simulink model "deneme"  (R2017b)
settings: Solver=ode45  StartTime=0.0  StopTime=10.0  MaxStep=1e-4  RelTol=1e-3
libraries: powerlib_extras x59, powerlib x57, powerlib_meascontrol x6, simulink x3, re_lib x3
(part 2 of 3)

== system deneme/Inverter Control/Current Ref. Generator ==
  note: evd
  note: evq
  evd : Inport
  evq : Inport  Port=2
  Divide : Product  Inputs=*/
  Divide1 : Product  Inputs=/*
  Scope24 : Scope
  Sum1 : Sum  Inputs=-+|
  Sum3 : Sum  Inputs=|++
  Zd : Gain  Gain=0.4559
  Zd1 : Gain  Gain=0.4559
  Zd^2+Zq^2 : Constant  Value=0.4559^2+0.1824^2
  Zq : Gain  Gain=0.1824
  Zq1 : Gain  Gain=0.1824
  id* : Outport
  iq* : Outport  Port=2
  tag scope: id_ref1=global, iq_ref1=global
  wires:
  Zd/1 -> Sum3/1
  Zq1/1 -> Sum3/2
  Zd1/1 -> Sum1/2
  Zq/1 -> Sum1/1
  Sum3/1 -> Divide/1
  Zd^2+Zq^2/1 -> Divide/2, Divide1/1, Scope24/1
  Sum1/1 -> Divide1/2
  evd/1 -> Zd/1, Zq/1
  evq/1 -> Zd1/1, Zq1/1
  Divide1/1 -> iq*/1, [iq_ref1]
  Divide/1 -> id*/1, [id_ref1]

== system deneme/Inverter Control/Frequency Reference Generator ==
  note: theta
  Constant : Constant  Value=2*pi
  Integrator : Integrator  ExternalReset=rising
  Relational Operator : RelationalOperator  OutDataTypeStr=boolean  RndMeth=Nearest
  "f* " : Constant  Value=50
  w* : Gain  Gain=2*pi
  theta* : Outport
  tag scope: f_ref=global, theta=global
  wires:
  "f* "/1 -> w*/1, [f_ref]
  w*/1 -> Integrator/1
  Relational Operator/1 -> Integrator/2
  Constant/1 -> Relational Operator/2
  Integrator/1 -> Relational Operator/1, theta*/1, [theta]

== system deneme/Inverter Control/Iabc  - idq ==
  Iabc : Inport
  theta : Inport  Port=2
  Demux : Demux  Outputs=2
  abc  - alfa/beta : Subsystem
  alfa/beta - dq : Subsystem
  iq : Outport
  id : Outport  Port=2
  tag scope: id1=global, iq1=global
  wires:
  theta/1 -> alfa/beta - dq/2(theta)
  Iabc/1 -> abc  - alfa/beta/1(abc)
  abc  - alfa/beta/1(alfa/beta) -> alfa/beta - dq/1(alfa/beta)
  alfa/beta - dq/1(d/q) -> Demux/1
  Demux/1 -> id/1, [id1]
  Demux/2 -> iq/1, [iq1]

== system deneme/Inverter Control/PI id ==
  e : Inport
  Gain1 : Gain  Gain=50
  Gain2 : Gain  Gain=500
  Integrator : Integrator
  Saturation : Saturate  UpperLimit=inf  LowerLimit=-inf
  Sum1 : Sum  Inputs=|++
  " " : Outport
  wires:
  Sum1/1 -> Saturation/1
  Integrator/1 -> Sum1/2
  Gain1/1 -> Sum1/1
  e/1 -> Gain2/1, Gain1/1
  Gain2/1 -> Integrator/1
  Saturation/1 -> " "/1

== system deneme/Inverter Control/PI iq ==
  e : Inport
  Gain1 : Gain  Gain=50
  Gain2 : Gain  Gain=500
  Integrator : Integrator
  Saturation : Saturate  UpperLimit=inf  LowerLimit=-inf
  Sum1 : Sum  Inputs=|++
  " " : Outport
  wires:
  Saturation/1 -> " "/1
  Gain2/1 -> Integrator/1
  e/1 -> Gain1/1, Gain2/1
  Gain1/1 -> Sum1/1
  Integrator/1 -> Sum1/2
  Sum1/1 -> Saturation/1

== system deneme/Inverter Control/PI vd ==
  e : Inport
  Gain1 : Gain  Gain=2
  Gain2 : Gain  Gain=20
  Integrator : Integrator
  Saturation : Saturate  UpperLimit=inf  LowerLimit=-inf
  Sum1 : Sum  Inputs=|++
  " " : Outport
  wires:
  Saturation/1 -> " "/1
  Gain2/1 -> Integrator/1
  e/1 -> Gain1/1, Gain2/1
  Gain1/1 -> Sum1/1
  Integrator/1 -> Sum1/2
  Sum1/1 -> Saturation/1

== system deneme/Inverter Control/PI vq ==
  e : Inport
  Gain1 : Gain  Gain=2
  Gain2 : Gain  Gain=2
  Integrator : Integrator
  Saturation : Saturate  UpperLimit=inf  LowerLimit=-inf
  Sum1 : Sum  Inputs=|++
  " " : Outport
  wires:
  Sum1/1 -> Saturation/1
  Integrator/1 -> Sum1/2
  Gain1/1 -> Sum1/1
  e/1 -> Gain2/1, Gain1/1
  Gain2/1 -> Integrator/1
  Saturation/1 -> " "/1

== system deneme/Inverter Control/PWM ==
  Uabc_ref : Inport
  Gain2 : Gain  Gain=2/1000
  PWM Generator : powerlib_extras/Control  Blocks/PWM Generator  GeneratorMode="3-arm  bridge (6 pulses)"  Fc=10000  Internal=off  mIndex=0.4  Freq=60  Phase=0
  S : Outport
  tag scope: m_index1=global, pulses1=global
  wires:
  PWM Generator/1 -> S/1, [pulses1]
  Uabc_ref/1 -> Gain2/1
  Gain2/1 -> PWM Generator/1, [m_index1]

== system deneme/Inverter Control/Vabc  - vdq ==
  Vabc : Inport
  theta : Inport  Port=2
  Demux : Demux  Outputs=2
  abc  - alfa/beta : Subsystem
  alfa/beta - dq : Subsystem
  vq : Outport
  vd : Outport  Port=2
  tag scope: vd1=global, vq1=global
  wires:
  Demux/2 -> vq/1, [vq1]
  Demux/1 -> vd/1, [vd1]
  alfa/beta - dq/1(d/q) -> Demux/1
  abc  - alfa/beta/1(alfa/beta) -> alfa/beta - dq/1(alfa/beta)
  Vabc/1 -> abc  - alfa/beta/1(abc)
  theta/1 -> alfa/beta - dq/2(theta)

== system deneme/Inverter Control/vdq - Vabc ==
  Ud/Uq : Inport
  theta : Inport  Port=2
  alfa/beta - abc : Subsystem
  d/q - alfa/beta : Subsystem
  Uabc_ref : Outport
  wires:
  d/q - alfa/beta/1(alfa/beta) -> alfa/beta - abc/1(alfa/beta)
  Ud/Uq/1 -> d/q - alfa/beta/1(d/q)
  alfa/beta - abc/1(abc) -> Uabc_ref/1
  theta/1 -> d/q - alfa/beta/2(tita)

== system deneme/Inverter Control1/ Voltage Reference Generator ==
  Mux4 : Mux  Inputs=3
  Phase A reference : Sin  Amplitude=400*sqrt(2)/sqrt(3)  Frequency=2*pi*50  SampleTime=0
  Phase B reference : Sin  Amplitude=400*sqrt(2)/sqrt(3)  Frequency=2*pi*50  Phase=-2*pi/3  SampleTime=0
  Phase C reference : Sin  Amplitude=400*sqrt(2)/sqrt(3)  Frequency=2*pi*50  Phase=2*pi/3  SampleTime=0
  Product : Product  RndMeth=Zero
  Ramp : simulink/Sources/Ramp  slope=1/0.3  start=0  X0=0
  Saturation : Saturate  UpperLimit=1  LowerLimit=0
  Vabc* : Outport
  tag scope: Vabc_ref2=global
  wires:
  Phase B reference/1 -> Mux4/2
  Phase A reference/1 -> Mux4/1
  Phase C reference/1 -> Mux4/3
  Ramp/1 -> Saturation/1
  Saturation/1 -> Product/2
  Mux4/1 -> Vabc*/1, [Vabc_ref2]

== system deneme/Inverter Control1/Cross Terms ==
  id* : Inport
  iq* : Inport  Port=2
  Gain1 : Gain  Gain=-2*pi*50*3e-3
  Gain2 : Gain  Gain=2*pi*50*3e-3
  " q" : Outport
  " d" : Outport  Port=2
  wires:
  id*/1 -> Gain1/1
  iq*/1 -> Gain2/1
  Gain1/1 -> " d"/1
  Gain2/1 -> " q"/1

== system deneme/Inverter Control1/Current Ref. Generator ==
  note: evd
  note: evq
  evd : Inport
  evq : Inport  Port=2
  Divide : Product  Inputs=*/
  Divide1 : Product  Inputs=/*
  Scope24 : Scope
  Sum1 : Sum  Inputs=-+|
  Sum3 : Sum  Inputs=|++
  Zd : Gain  Gain=0.4559
  Zd1 : Gain  Gain=0.4559
  Zd^2+Zq^2 : Constant  Value=0.4559^2+0.1824^2
  Zq : Gain  Gain=0.1824
  Zq1 : Gain  Gain=0.1824
  id* : Outport
  iq* : Outport  Port=2
  tag scope: id_ref2=global, iq_ref2=global
  wires:
  Zd/1 -> Sum3/1
  Zq1/1 -> Sum3/2
  Zd1/1 -> Sum1/2
  Zq/1 -> Sum1/1
  Sum3/1 -> Divide/1
  Zd^2+Zq^2/1 -> Divide/2, Divide1/1, Scope24/1
  Sum1/1 -> Divide1/2
  evd/1 -> Zd/1, Zq/1
  evq/1 -> Zd1/1, Zq1/1
  Divide1/1 -> iq*/1, [iq_ref2]
  Divide/1 -> id*/1, [id_ref2]

== system deneme/Inverter Control1/Frequency Reference Generator ==
  note: theta
  Constant : Constant  Value=2*pi
  Integrator : Integrator  ExternalReset=rising
  Relational Operator : RelationalOperator  OutDataTypeStr=boolean  RndMeth=Nearest
  "f* " : Constant  Value=50
  w* : Gain  Gain=2*pi
  theta* : Outport
  wires:
  "f* "/1 -> w*/1
  w*/1 -> Integrator/1
  Relational Operator/1 -> Integrator/2
  Constant/1 -> Relational Operator/2
  Integrator/1 -> Relational Operator/1, theta*/1

== system deneme/Inverter Control1/Iabc  - idq ==
  Iabc : Inport
  theta : Inport  Port=2
  Demux : Demux  Outputs=2
  abc  - alfa/beta : Subsystem
  alfa/beta - dq : Subsystem
  iq : Outport
  id : Outport  Port=2
  tag scope: id2=global, iq2=global
  wires:
  theta/1 -> alfa/beta - dq/2(theta)
  Iabc/1 -> abc  - alfa/beta/1(abc)
  abc  - alfa/beta/1(alfa/beta) -> alfa/beta - dq/1(alfa/beta)
  alfa/beta - dq/1(d/q) -> Demux/1
  Demux/1 -> id/1, [id2]
  Demux/2 -> iq/1, [iq2]

== system deneme/Inverter Control1/PI id ==
  e : Inport
  Gain1 : Gain  Gain=50
  Gain2 : Gain  Gain=500
  Integrator : Integrator
  Saturation : Saturate  UpperLimit=inf  LowerLimit=-inf
  Sum1 : Sum  Inputs=|++
  " " : Outport
  wires:
  Sum1/1 -> Saturation/1
  Integrator/1 -> Sum1/2
  Gain1/1 -> Sum1/1
  e/1 -> Gain2/1, Gain1/1
  Gain2/1 -> Integrator/1
  Saturation/1 -> " "/1

== system deneme/Inverter Control1/PI iq ==
  e : Inport
  Gain1 : Gain  Gain=50
  Gain2 : Gain  Gain=500
  Integrator : Integrator
  Saturation : Saturate  UpperLimit=inf  LowerLimit=-inf
  Sum1 : Sum  Inputs=|++
  " " : Outport
  wires:
  Saturation/1 -> " "/1
  Gain2/1 -> Integrator/1
  e/1 -> Gain1/1, Gain2/1
  Gain1/1 -> Sum1/1
  Integrator/1 -> Sum1/2
  Sum1/1 -> Saturation/1

== system deneme/Inverter Control1/PI vd ==
  e : Inport
  Gain1 : Gain  Gain=2
  Gain2 : Gain  Gain=20
  Integrator : Integrator
  Saturation : Saturate  UpperLimit=inf  LowerLimit=-inf
  Sum1 : Sum  Inputs=|++
  " " : Outport
  wires:
  Saturation/1 -> " "/1
  Gain2/1 -> Integrator/1
  e/1 -> Gain1/1, Gain2/1
  Gain1/1 -> Sum1/1
  Integrator/1 -> Sum1/2
  Sum1/1 -> Saturation/1

== system deneme/Inverter Control1/PI vq ==
  e : Inport
  Gain1 : Gain  Gain=2
  Gain2 : Gain  Gain=2
  Integrator : Integrator
  Saturation : Saturate  UpperLimit=inf  LowerLimit=-inf
  Sum1 : Sum  Inputs=|++
  " " : Outport
  wires:
  Sum1/1 -> Saturation/1
  Integrator/1 -> Sum1/2
  Gain1/1 -> Sum1/1
  e/1 -> Gain2/1, Gain1/1
  Gain2/1 -> Integrator/1
  Saturation/1 -> " "/1

== system deneme/Inverter Control1/PWM ==
  Uabc_ref : Inport
  Gain2 : Gain  Gain=2/1000
  PWM Generator : powerlib_extras/Control  Blocks/PWM Generator  GeneratorMode="3-arm  bridge (6 pulses)"  Fc=10000  Internal=off  mIndex=0.4  Freq=60  Phase=0
  S : Outport
  tag scope: m_index2=global, pulses2=global
  wires:
  PWM Generator/1 -> S/1, [pulses2]
  Uabc_ref/1 -> Gain2/1
  Gain2/1 -> PWM Generator/1, [m_index2]

== system deneme/Inverter Control1/Vabc  - vdq ==
  Vabc : Inport
  theta : Inport  Port=2
  Demux : Demux  Outputs=2
  abc  - alfa/beta : Subsystem
  alfa/beta - dq : Subsystem
  vq : Outport
  vd : Outport  Port=2
  tag scope: vd2=global, vq2=global
  wires:
  Demux/2 -> vq/1, [vq2]
  Demux/1 -> vd/1, [vd2]
  alfa/beta - dq/1(d/q) -> Demux/1
  abc  - alfa/beta/1(alfa/beta) -> alfa/beta - dq/1(alfa/beta)
  Vabc/1 -> abc  - alfa/beta/1(abc)
  theta/1 -> alfa/beta - dq/2(theta)

== system deneme/Inverter Control1/vdq - Vabc ==
  Ud/Uq : Inport
  theta : Inport  Port=2
  alfa/beta - abc : Subsystem
  d/q - alfa/beta : Subsystem
  Uabc_ref : Outport
  wires:
  d/q - alfa/beta/1(alfa/beta) -> alfa/beta - abc/1(alfa/beta)
  Ud/Uq/1 -> d/q - alfa/beta/1(d/q)
  alfa/beta - abc/1(abc) -> Uabc_ref/1
  theta/1 -> d/q - alfa/beta/2(tita)

== system deneme/Inverter Control2/ Voltage Reference Generator ==
  Mux4 : Mux  Inputs=3
  Phase A reference : Sin  Amplitude=400*sqrt(2)/sqrt(3)  Frequency=2*pi*50  SampleTime=0
  Phase B reference : Sin  Amplitude=400*sqrt(2)/sqrt(3)  Frequency=2*pi*50  Phase=-2*pi/3  SampleTime=0
  Phase C reference : Sin  Amplitude=400*sqrt(2)/sqrt(3)  Frequency=2*pi*50  Phase=2*pi/3  SampleTime=0
  Product : Product  RndMeth=Zero
  Ramp : simulink/Sources/Ramp  slope=1/0.3  start=0  X0=0
  Saturation : Saturate  UpperLimit=1  LowerLimit=0
  Vabc* : Outport
  tag scope: Vabc_ref3=global
  wires:
  Phase B reference/1 -> Mux4/2
  Phase A reference/1 -> Mux4/1
  Phase C reference/1 -> Mux4/3
  Ramp/1 -> Saturation/1
  Saturation/1 -> Product/2
  Mux4/1 -> Vabc*/1, [Vabc_ref3]

== system deneme/Inverter Control2/Cross Terms ==
  id* : Inport
  iq* : Inport  Port=2
  Gain1 : Gain  Gain=-2*pi*50*3e-3
  Gain2 : Gain  Gain=2*pi*50*3e-3
  " q" : Outport
  " d" : Outport  Port=2
  wires:
  id*/1 -> Gain1/1
  iq*/1 -> Gain2/1
  Gain1/1 -> " d"/1
  Gain2/1 -> " q"/1

== system deneme/Inverter Control2/Current Ref. Generator ==
  note: evd
  note: evq
  evd : Inport
  evq : Inport  Port=2
  Divide : Product  Inputs=*/
  Divide1 : Product  Inputs=/*
  Scope24 : Scope
  Sum1 : Sum  Inputs=-+|
  Sum3 : Sum  Inputs=|++
  Zd : Gain  Gain=0.4559
  Zd1 : Gain  Gain=0.4559
  Zd^2+Zq^2 : Constant  Value=0.4559^2+0.1824^2
  Zq : Gain  Gain=0.1824
  Zq1 : Gain  Gain=0.1824
  id* : Outport
  iq* : Outport  Port=2
  tag scope: id_ref3=global, iq_ref3=global
  wires:
  Zd/1 -> Sum3/1
  Zq1/1 -> Sum3/2
  Zd1/1 -> Sum1/2
  Zq/1 -> Sum1/1
  Sum3/1 -> Divide/1
  Zd^2+Zq^2/1 -> Divide/2, Divide1/1, Scope24/1
  Sum1/1 -> Divide1/2
  evd/1 -> Zd/1, Zq/1
  evq/1 -> Zd1/1, Zq1/1
  Divide1/1 -> iq*/1, [iq_ref3]
  Divide/1 -> id*/1, [id_ref3]

== system deneme/Inverter Control2/Frequency Reference Generator ==
  note: theta
  Constant : Constant  Value=2*pi
  Integrator : Integrator  ExternalReset=rising
  Relational Operator : RelationalOperator  OutDataTypeStr=boolean  RndMeth=Nearest
  "f* " : Constant  Value=50
  w* : Gain  Gain=2*pi
  theta* : Outport
  wires:
  "f* "/1 -> w*/1
  w*/1 -> Integrator/1
  Relational Operator/1 -> Integrator/2
  Constant/1 -> Relational Operator/2
  Integrator/1 -> Relational Operator/1, theta*/1

== system deneme/Inverter Control2/Iabc  - idq ==
  Iabc : Inport
  theta : Inport  Port=2
  Demux : Demux  Outputs=2
  abc  - alfa/beta : Subsystem
  alfa/beta - dq : Subsystem
  iq : Outport
  id : Outport  Port=2
  tag scope: id3=global, iq3=global
  wires:
  theta/1 -> alfa/beta - dq/2(theta)
  Iabc/1 -> abc  - alfa/beta/1(abc)
  abc  - alfa/beta/1(alfa/beta) -> alfa/beta - dq/1(alfa/beta)
  alfa/beta - dq/1(d/q) -> Demux/1
  Demux/1 -> id/1, [id3]
  Demux/2 -> iq/1, [iq3]

== system deneme/Inverter Control2/PI id ==
  e : Inport
  Gain1 : Gain  Gain=50
  Gain2 : Gain  Gain=500
  Integrator : Integrator
  Saturation : Saturate  UpperLimit=inf  LowerLimit=-inf
  Sum1 : Sum  Inputs=|++
  " " : Outport
  wires:
  Sum1/1 -> Saturation/1
  Integrator/1 -> Sum1/2
  Gain1/1 -> Sum1/1
  e/1 -> Gain2/1, Gain1/1
  Gain2/1 -> Integrator/1
  Saturation/1 -> " "/1

== system deneme/Inverter Control2/PI iq ==
  e : Inport
  Gain1 : Gain  Gain=50
  Gain2 : Gain  Gain=500
  Integrator : Integrator
  Saturation : Saturate  UpperLimit=inf  LowerLimit=-inf
  Sum1 : Sum  Inputs=|++
  " " : Outport
  wires:
  Saturation/1 -> " "/1
  Gain2/1 -> Integrator/1
  e/1 -> Gain1/1, Gain2/1
  Gain1/1 -> Sum1/1
  Integrator/1 -> Sum1/2
  Sum1/1 -> Saturation/1

== system deneme/Inverter Control2/PI vd ==
  e : Inport
  Gain1 : Gain  Gain=2
  Gain2 : Gain  Gain=20
  Integrator : Integrator
  Saturation : Saturate  UpperLimit=inf  LowerLimit=-inf
  Sum1 : Sum  Inputs=|++
  " " : Outport
  wires:
  Saturation/1 -> " "/1
  Gain2/1 -> Integrator/1
  e/1 -> Gain1/1, Gain2/1
  Gain1/1 -> Sum1/1
  Integrator/1 -> Sum1/2
  Sum1/1 -> Saturation/1

== system deneme/Inverter Control2/PI vq ==
  e : Inport
  Gain1 : Gain  Gain=2
  Gain2 : Gain  Gain=2
  Integrator : Integrator
  Saturation : Saturate  UpperLimit=inf  LowerLimit=-inf
  Sum1 : Sum  Inputs=|++
  " " : Outport
  wires:
  Sum1/1 -> Saturation/1
  Integrator/1 -> Sum1/2
  Gain1/1 -> Sum1/1
  e/1 -> Gain2/1, Gain1/1
  Gain2/1 -> Integrator/1
  Saturation/1 -> " "/1

== system deneme/Inverter Control2/PWM ==
  Uabc_ref : Inport
  Gain2 : Gain  Gain=2/1000
  PWM Generator : powerlib_extras/Control  Blocks/PWM Generator  GeneratorMode="3-arm  bridge (6 pulses)"  Fc=10000  Internal=off  mIndex=0.4  Freq=60  Phase=0
  S : Outport
  tag scope: m_index3=global, pulses3=global
  wires:
  PWM Generator/1 -> S/1, [pulses3]
  Uabc_ref/1 -> Gain2/1
  Gain2/1 -> PWM Generator/1, [m_index3]

== system deneme/Inverter Control2/Vabc  - vdq ==
  Vabc : Inport
  theta : Inport  Port=2
  Demux : Demux  Outputs=2
  abc  - alfa/beta : Subsystem
  alfa/beta - dq : Subsystem
  vq : Outport
  vd : Outport  Port=2
  tag scope: vd3=global, vq3=global
  wires:
  Demux/2 -> vq/1, [vq3]
  Demux/1 -> vd/1, [vd3]
  alfa/beta - dq/1(d/q) -> Demux/1
  abc  - alfa/beta/1(alfa/beta) -> alfa/beta - dq/1(alfa/beta)
  Vabc/1 -> abc  - alfa/beta/1(abc)
  theta/1 -> alfa/beta - dq/2(theta)

== system deneme/Inverter Control2/vdq - Vabc ==
  Ud/Uq : Inport
  theta : Inport  Port=2
  alfa/beta - abc : Subsystem
  d/q - alfa/beta : Subsystem
  Uabc_ref : Outport
  wires:
  d/q - alfa/beta/1(alfa/beta) -> alfa/beta - abc/1(alfa/beta)
  Ud/Uq/1 -> d/q - alfa/beta/1(d/q)
  alfa/beta - abc/1(abc) -> Uabc_ref/1
  theta/1 -> d/q - alfa/beta/2(tita)

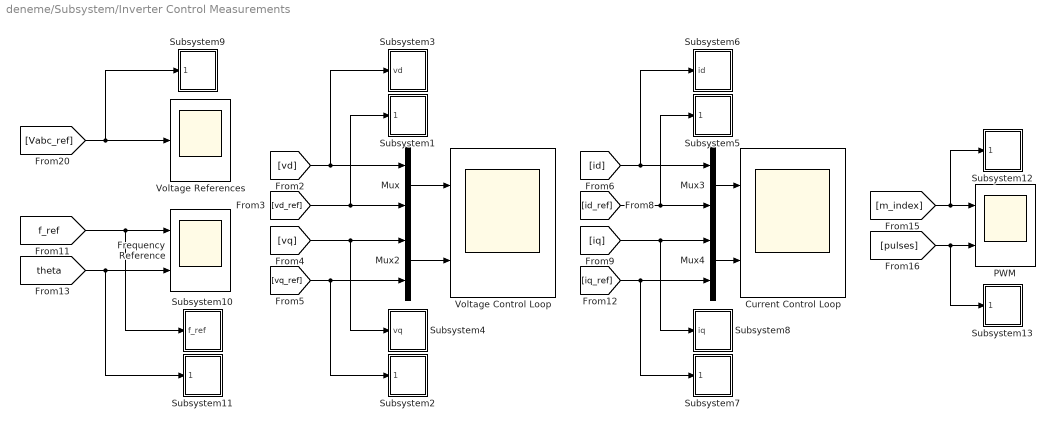
== system deneme/Subsystem/Inverter Control Measurements ==
  Current Control Loop : Scope  NumInputPorts=2
  Frequency Reference : Scope  NumInputPorts=2
  Mux{,2..4} (4 alike) : Mux  Inputs=2
  PWM : Scope  NumInputPorts=2
  Subsystem1 : Subsystem
  Subsystem10 : Subsystem
  Subsystem11 : Subsystem
  Subsystem12 : Subsystem
  Subsystem13 : Subsystem
  Subsystem2 : Subsystem
  Subsystem3 : Subsystem
  Subsystem4 : Subsystem
  Subsystem5 : Subsystem
  Subsystem6 : Subsystem
  Subsystem7 : Subsystem
  Subsystem8 : Subsystem
  Subsystem9 : Subsystem
  Voltage Control Loop : Scope  NumInputPorts=2
  Voltage References : Scope
  wires:
  [vd] -> Mux/1, Subsystem3/1(vd)
  [vd_ref] -> Mux/2, Subsystem1/1(vd_ref)
  [vq] -> Mux2/1, Subsystem4/1(vq)
  [vq_ref] -> Mux2/2, Subsystem2/1(vq_ref)
  Mux/1 -> Voltage Control Loop/1
  Mux2/1 -> Voltage Control Loop/2
  [id] -> Mux3/1, Subsystem6/1(id)
  [id_ref] -> Mux3/2, Subsystem5/1(id_ref)
  [iq] -> Mux4/1, Subsystem8/1(iq)
  [iq_ref] -> Mux4/2, Subsystem7/1(iq_ref)
  [Vabc_ref] -> Voltage References/1, Subsystem9/1(Vabc_ref)
  Mux3/1 -> Current Control Loop/1
  Mux4/1 -> Current Control Loop/2
  [theta] -> Frequency Reference/2, Subsystem11/1(theta)
  [f_ref] -> Frequency Reference/1, Subsystem10/1(f_ref)
  [pulses] -> PWM/2, Subsystem13/1(pulses)
  [m_index] -> PWM/1, Subsystem12/1(m_index)

== system deneme/Subsystem/Inverter Control Measurements1 ==
  Boost Converter Control MPPT : Scope  NumInputPorts=3
  wires:
  [Vref] -> Boost Converter Control MPPT/1
  [delta] -> Boost Converter Control MPPT/2
  [pulsos] -> Boost Converter Control MPPT/3

== system deneme/Subsystem/Inverter Control Measurements2 ==
  Control Loops : Scope  NumInputPorts=2
  Mux : Mux  Inputs=2
  Mux2 : Mux  Inputs=2
  Switch Control : Scope  NumInputPorts=3
  wires:
  [Vdc] -> Mux/1
  [Vdc_ref] -> Mux/2
  [Ibat] -> Mux2/1
  [Ibat_ref] -> Mux2/2
  Mux/1 -> Control Loops/1
  Mux2/1 -> Control Loops/2
  [Sign] -> Switch Control/1
  [S1] -> Switch Control/2
  [S2] -> Switch Control/3

== system deneme/Subsystem/Inverter Control Measurements3 ==
  PLL : Subsystem
  Subsystem : Subsystem
  wires:
  Subsystem/1(Vabc) -> PLL/1(Vabc)

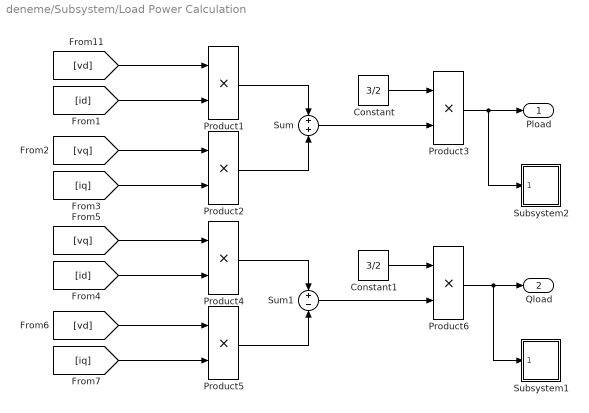
== system deneme/Subsystem/Load Power Calculation ==
  Constant : Constant  Value=3/2
  Constant1 : Constant  Value=3/2
  Product{1..6} (6 alike) : Product  RndMeth=Zero
  Subsystem1 : Subsystem
  Subsystem2 : Subsystem
  Sum : Sum  Inputs=+|+
  Sum1 : Sum  Inputs=+|-
  Pload : Outport
  Qload : Outport  Port=2
  wires:
  [vd] -> Product1/1
  [id] -> Product1/2
  [vq] -> Product2/1
  [iq] -> Product2/2
  Product1/1 -> Sum/1
  Product2/1 -> Sum/2
  Sum/1 -> Product3/2
  Constant/1 -> Product3/1
  Product3/1 -> Pload/1, Subsystem2/1(Pload)
  [vq] -> Product4/1
  [id] -> Product4/2
  [vd] -> Product5/1
  [iq] -> Product5/2
  Product4/1 -> Sum1/1
  Product5/1 -> Sum1/2
  Sum1/1 -> Product6/2
  Constant1/1 -> Product6/1
  Product6/1 -> Qload/1, Subsystem1/1(Qacload)

== system deneme/Subsystem/Subsystem ==
  Mux : Mux  Inputs=3
  Vabc : Outport
  wires:
  Mux/1 -> Vabc/1
  [Vab] -> Mux/1
  [Vbc] -> Mux/2
  [Vca] -> Mux/3

== system deneme/Subsystem/Subsystem1 ==
  Pbus : Inport
  LPF vq11 : powerlib_extras/Discrete  Control Blocks/Discrete 1st-Order Filter  FilterType=Lowpass  Tc=10e-3  Ts=5e-6  Initialize=off  Vac_Init=[0.8 -25 60]  Vdc_Init=0  PlotResponse=off  param1=[1 100 0.1]
  To Workspace1 : ToWorkspace  VariableName=Pbus  SampleTime=-1
  To Workspace2 : ToWorkspace  VariableName=Pbus1  SampleTime=-1
  tag scope: Pbus=global
  wires:
  Pbus/1 -> [Pbus], To Workspace1/1, LPF vq11/1
  LPF vq11/1 -> To Workspace2/1

== system deneme/Subsystem/Subsystem10 ==
  f : Inport
  LPF vq7 : powerlib_extras/Discrete  Control Blocks/Discrete 1st-Order Filter  FilterType=Lowpass  Tc=10e-3  Ts=5e-6  Initialize=off  Vac_Init=[0.8 -25 60]  Vdc_Init=0  PlotResponse=off  param1=[1 100 0.1]
  To Workspace1 : ToWorkspace  VariableName=fabc_real  SampleTime=-1
  To Workspace2 : ToWorkspace  VariableName=fabc_real_fil  SampleTime=-1
  Zero-Order Hold : ZeroOrderHold  SampleTime=5e-6
  wires:
  f/1 -> Zero-Order Hold/1
  LPF vq7/1 -> To Workspace2/1
  Zero-Order Hold/1 -> To Workspace1/1, LPF vq7/1

== system deneme/Subsystem/Subsystem11 ==
  LPF vq{2..3,8..9} (4 alike) : powerlib_extras/Discrete  Control Blocks/Discrete 1st-Order Filter  FilterType=Lowpass  Tc=10e-3  Ts=5e-6  Initialize=off  Vac_Init=[0.8 -25 60]  Vdc_Init=0  PlotResponse=off  param1=[1 100 0.1]
  Load Measurements1 : Scope  NumInputPorts=2
  Load Measurements3 : Scope  NumInputPorts=2
  Load Power Calculation1 : Subsystem
  Load Power Calculation2 : Subsystem
  Load Powers1 : Scope  NumInputPorts=2
  Load Powers2 : Scope  NumInputPorts=2
  wires:
  [Vabc2] -> Load Measurements1/1
  [Iabc2] -> Load Measurements1/2
  Load Power Calculation1/1(Pload) -> LPF vq2/1
  Load Power Calculation1/2(Qload) -> LPF vq3/1
  LPF vq2/1 -> Load Powers1/1
  LPF vq3/1 -> Load Powers1/2
  [Vabc3] -> Load Measurements3/1
  [Iabc3] -> Load Measurements3/2
  Load Power Calculation2/1(Pload) -> LPF vq8/1
  Load Power Calculation2/2(Qload) -> LPF vq9/1
  LPF vq8/1 -> Load Powers2/1
  LPF vq9/1 -> Load Powers2/2

== system deneme/Subsystem/Subsystem3 ==
  Pdc : Inport
  LPF vq7 : powerlib_extras/Discrete  Control Blocks/Discrete 1st-Order Filter  FilterType=Lowpass  Tc=10e-3  Ts=5e-6  Initialize=off  Vac_Init=[0.8 -25 60]  Vdc_Init=0  PlotResponse=off  param1=[1 100 0.1]
  To Workspace1 : ToWorkspace  VariableName=Pdc  SampleTime=-1
  To Workspace2 : ToWorkspace  VariableName=Pdc1  SampleTime=-1
  tag scope: Pdc=global
  wires:
  Pdc/1 -> [Pdc], To Workspace1/1, LPF vq7/1
  LPF vq7/1 -> To Workspace2/1

== system deneme/Subsystem/Subsystem4 ==
  Ppv : Inport
  LPF vq7 : powerlib_extras/Discrete  Control Blocks/Discrete 1st-Order Filter  FilterType=Lowpass  Tc=10e-3  Ts=5e-6  Initialize=off  Vac_Init=[0.8 -25 60]  Vdc_Init=0  PlotResponse=off  param1=[1 100 0.1]
  To Workspace1 : ToWorkspace  VariableName=Ppv  SampleTime=-1
  To Workspace2 : ToWorkspace  VariableName=Ppv1  SampleTime=-1
  tag scope: Ppv=global
  wires:
  Ppv/1 -> [Ppv], To Workspace1/1, LPF vq7/1
  LPF vq7/1 -> To Workspace2/1

== system deneme/Subsystem/Subsystem5 ==
  Pbat : Inport
  LPF vq7 : powerlib_extras/Discrete  Control Blocks/Discrete 1st-Order Filter  FilterType=Lowpass  Tc=10e-3  Ts=5e-6  Initialize=off  Vac_Init=[0.8 -25 60]  Vdc_Init=0  PlotResponse=off  param1=[1 100 0.1]
  To Workspace1 : ToWorkspace  VariableName=Pbat  SampleTime=-1
  To Workspace2 : ToWorkspace  VariableName=Pbat1  SampleTime=-1
  tag scope: Pbat=global
  wires:
  Pbat/1 -> [Pbat], To Workspace1/1, LPF vq7/1
  LPF vq7/1 -> To Workspace2/1

== system deneme/Subsystem/Subsystem6 ==
  Vab_rms : Inport
  To Workspace1 : ToWorkspace  VariableName=Vab_rms  SampleTime=-1
  tag scope: Vab_rms=global
  wires:
  Vab_rms/1 -> To Workspace1/1, [Vab_rms]

== system deneme/Subsystem/Subsystem7 ==
  Va_rms : Inport
  To Workspace1 : ToWorkspace  VariableName=Va_rms  SampleTime=-1
  tag scope: Va_rms=global
  wires:
  Va_rms/1 -> [Va_rms], To Workspace1/1

== system deneme/Subsystem/Subsystem8 ==
  Pdcinv : Inport
  LPF vq7 : powerlib_extras/Discrete  Control Blocks/Discrete 1st-Order Filter  FilterType=Lowpass  Tc=10e-3  Ts=5e-6  Initialize=off  Vac_Init=[0.8 -25 60]  Vdc_Init=0  PlotResponse=off  param1=[1 100 0.1]
  To Workspace1 : ToWorkspace  VariableName=Pdcinv  SampleTime=-1
  To Workspace2 : ToWorkspace  VariableName=Pdcinv1  SampleTime=-1
  tag scope: Pdcinv=global
  wires:
  Pdcinv/1 -> [Pdcinv], To Workspace1/1, LPF vq7/1
  LPF vq7/1 -> To Workspace2/1

== system deneme/Subsystem/Subsystem9 ==
  Mux1 : Mux  Inputs=3
  Iabc : Outport
  wires:
  [Ia] -> Mux1/1
  [Ib] -> Mux1/2
  [Ic] -> Mux1/3
  Mux1/1 -> Iabc/1

== system deneme/Boost/Incremental Conductance MPPT/Subsystem1 ==
  Vref : Inport
  To Workspace1 : ToWorkspace  VariableName=Vref  SampleTime=-1
  Zero-Order Hold : ZeroOrderHold  SampleTime=5e-6
  tag scope: Vref=global
  wires:
  Vref/1 -> Zero-Order Hold/1
  Zero-Order Hold/1 -> [Vref], To Workspace1/1

== system deneme/Boost/Incremental Conductance MPPT/Subsystem2 ==
  delta : Inport
  To Workspace1 : ToWorkspace  VariableName=delta  SampleTime=-1
  Zero-Order Hold : ZeroOrderHold  SampleTime=5e-6
  tag scope: delta=global
  wires:
  delta/1 -> Zero-Order Hold/1
  Zero-Order Hold/1 -> To Workspace1/1, [delta]

== system deneme/Boost/Incremental Conductance MPPT/Subsystem3 ==
  pulsos : Inport
  To Workspace1 : ToWorkspace  VariableName=pulsos  SampleTime=-1
  Zero-Order Hold : ZeroOrderHold  SampleTime=5e-6
  tag scope: pulsos=global
  wires:
  pulsos/1 -> Zero-Order Hold/1
  Zero-Order Hold/1 -> [pulsos], To Workspace1/1

== system deneme/Boost1/Incremental Conductance MPPT/Subsystem1 ==
  Vref : Inport
  To Workspace1 : ToWorkspace  VariableName=Vref2  SampleTime=-1
  Zero-Order Hold : ZeroOrderHold  SampleTime=5e-6
  tag scope: Vref2=global
  wires:
  Vref/1 -> Zero-Order Hold/1
  Zero-Order Hold/1 -> To Workspace1/1, [Vref2]

== system deneme/Boost1/Incremental Conductance MPPT/Subsystem2 ==
  delta : Inport
  To Workspace1 : ToWorkspace  VariableName=delta2  SampleTime=-1
  Zero-Order Hold : ZeroOrderHold  SampleTime=5e-6
  tag scope: delta2=global
  wires:
  delta/1 -> Zero-Order Hold/1
  Zero-Order Hold/1 -> To Workspace1/1, [delta2]

== system deneme/Boost1/Incremental Conductance MPPT/Subsystem3 ==
  pulsos : Inport
  To Workspace1 : ToWorkspace  VariableName=pulsos2  SampleTime=-1
  Zero-Order Hold : ZeroOrderHold  SampleTime=5e-6
  tag scope: pulsos2=global
  wires:
  pulsos/1 -> Zero-Order Hold/1
  Zero-Order Hold/1 -> [pulsos2], To Workspace1/1

== system deneme/Boost2/Incremental Conductance MPPT/Subsystem1 ==
  Vref : Inport
  To Workspace1 : ToWorkspace  VariableName=Vref3  SampleTime=-1
  Zero-Order Hold : ZeroOrderHold  SampleTime=5e-6
  tag scope: Vref3=global
  wires:
  Zero-Order Hold/1 -> [Vref3], To Workspace1/1
  Vref/1 -> Zero-Order Hold/1

== system deneme/Boost2/Incremental Conductance MPPT/Subsystem2 ==
  delta : Inport
  To Workspace1 : ToWorkspace  VariableName=delta3  SampleTime=-1
  Zero-Order Hold : ZeroOrderHold  SampleTime=5e-6
  tag scope: delta3=global
  wires:
  Zero-Order Hold/1 -> [delta3], To Workspace1/1
  delta/1 -> Zero-Order Hold/1

== system deneme/Boost2/Incremental Conductance MPPT/Subsystem3 ==
  pulsos : Inport
  To Workspace1 : ToWorkspace  VariableName=pulsos3  SampleTime=-1
  Zero-Order Hold : ZeroOrderHold  SampleTime=5e-6
  tag scope: pulsos3=global
  wires:
  Zero-Order Hold/1 -> To Workspace1/1, [pulsos3]
  pulsos/1 -> Zero-Order Hold/1

== system deneme/Inverter Control/Iabc  - idq/abc  - alfa//beta ==
  abc : Inport
  Mux : Mux  Inputs=2
  d_s : Fcn  Expr=(-1/sqrt(3)*u(2))+(1/sqrt(3)*u(3))
  q_s : Fcn  Expr=(2/3)*u(1)-(1/3)*u(2)-(1/3)*u(3)
  alfa/beta : Outport
  wires:
  abc/1 -> q_s/1, d_s/1
  d_s/1 -> Mux/1
  q_s/1 -> Mux/2
  Mux/1 -> alfa/beta/1

== system deneme/Inverter Control/Iabc  - idq/alfa//beta - dq ==
  alfa/beta : Inport
  theta : Inport  Port=2
  Mux : Mux  Inputs=2
  Mux1 : Mux  Inputs=2
  d : Fcn  Expr=u(2)*sin(u(3)) + u(1)*cos(u(3))
  q : Fcn  Expr=-u(1)*sin(u(3)) + u(2)*cos(u(3))
  d/q : Outport
  wires:
  d/1 -> Mux/1
  q/1 -> Mux/2
  Mux/1 -> d/q/1
  alfa/beta/1 -> Mux1/1
  theta/1 -> Mux1/2
  Mux1/1 -> d/1, q/1

== system deneme/Inverter Control/Vabc  - vdq/abc  - alfa//beta ==
  abc : Inport
  Mux : Mux  Inputs=2
  d_s : Fcn  Expr=(-1/sqrt(3)*u(2))+(1/sqrt(3)*u(3))
  q_s : Fcn  Expr=(2/3)*u(1)-(1/3)*u(2)-(1/3)*u(3)
  alfa/beta : Outport
  wires:
  Mux/1 -> alfa/beta/1
  q_s/1 -> Mux/2
  d_s/1 -> Mux/1
  abc/1 -> d_s/1, q_s/1

== system deneme/Inverter Control/Vabc  - vdq/alfa//beta - dq ==
  alfa/beta : Inport
  theta : Inport  Port=2
  Mux : Mux  Inputs=2
  Mux1 : Mux  Inputs=2
  d : Fcn  Expr=u(2)*sin(u(3)) + u(1)*cos(u(3))
  q : Fcn  Expr=-u(1)*sin(u(3)) + u(2)*cos(u(3))
  d/q : Outport
  wires:
  Mux1/1 -> q/1, d/1
  theta/1 -> Mux1/2
  alfa/beta/1 -> Mux1/1
  Mux/1 -> d/q/1
  q/1 -> Mux/2
  d/1 -> Mux/1

== system deneme/Inverter Control/vdq - Vabc/alfa//beta - abc ==
  alfa/beta : Inport
  Mux : Mux  Inputs=3
  a : Fcn  Expr=u[2]
  b : Fcn  Expr=-sqrt(3)/2*u[1]-0.5*u[2]
  c : Fcn  Expr=sqrt(3)/2*u[1]-0.5*u[2]
  abc : Outport
  tag scope: Vca_ref1=global, Vcb_ref1=global, Vcc_ref1=global
  wires:
  alfa/beta/1 -> c/1, a/1, b/1
  Mux/1 -> abc/1
  c/1 -> Mux/3, [Vcc_ref1]
  b/1 -> Mux/2, [Vcb_ref1]
  a/1 -> Mux/1, [Vca_ref1]

== system deneme/Inverter Control/vdq - Vabc/d//q - alfa//beta ==
  d/q : Inport
  tita : Inport  Port=2
  Mux : Mux  Inputs=2
  Mux1 : Mux  Inputs=2
  a : Fcn  Expr=-u[2]*sin(u[3]) + u[1]*cos(u[3])
  b : Fcn  Expr=u[1]*sin(u[3]) + u[2]*cos(u[3])
  alfa/beta : Outport
  wires:
  Mux1/1 -> b/1, a/1
  tita/1 -> Mux1/2
  d/q/1 -> Mux1/1
  a/1 -> Mux/1
  b/1 -> Mux/2
  Mux/1 -> alfa/beta/1

== system deneme/Inverter Control1/Iabc  - idq/abc  - alfa//beta ==
  abc : Inport
  Mux : Mux  Inputs=2
  d_s : Fcn  Expr=(-1/sqrt(3)*u(2))+(1/sqrt(3)*u(3))
  q_s : Fcn  Expr=(2/3)*u(1)-(1/3)*u(2)-(1/3)*u(3)
  alfa/beta : Outport
  wires:
  abc/1 -> q_s/1, d_s/1
  d_s/1 -> Mux/1
  q_s/1 -> Mux/2
  Mux/1 -> alfa/beta/1

== system deneme/Inverter Control1/Iabc  - idq/alfa//beta - dq ==
  alfa/beta : Inport
  theta : Inport  Port=2
  Mux : Mux  Inputs=2
  Mux1 : Mux  Inputs=2
  d : Fcn  Expr=u(2)*sin(u(3)) + u(1)*cos(u(3))
  q : Fcn  Expr=-u(1)*sin(u(3)) + u(2)*cos(u(3))
  d/q : Outport
  wires:
  d/1 -> Mux/1
  q/1 -> Mux/2
  Mux/1 -> d/q/1
  alfa/beta/1 -> Mux1/1
  theta/1 -> Mux1/2
  Mux1/1 -> d/1, q/1

== system deneme/Inverter Control1/Vabc  - vdq/abc  - alfa//beta ==
  abc : Inport
  Mux : Mux  Inputs=2
  d_s : Fcn  Expr=(-1/sqrt(3)*u(2))+(1/sqrt(3)*u(3))
  q_s : Fcn  Expr=(2/3)*u(1)-(1/3)*u(2)-(1/3)*u(3)
  alfa/beta : Outport
  wires:
  Mux/1 -> alfa/beta/1
  q_s/1 -> Mux/2
  d_s/1 -> Mux/1
  abc/1 -> d_s/1, q_s/1

== system deneme/Inverter Control1/Vabc  - vdq/alfa//beta - dq ==
  alfa/beta : Inport
  theta : Inport  Port=2
  Mux : Mux  Inputs=2
  Mux1 : Mux  Inputs=2
  d : Fcn  Expr=u(2)*sin(u(3)) + u(1)*cos(u(3))
  q : Fcn  Expr=-u(1)*sin(u(3)) + u(2)*cos(u(3))
  d/q : Outport
  wires:
  Mux1/1 -> q/1, d/1
  theta/1 -> Mux1/2
  alfa/beta/1 -> Mux1/1
  Mux/1 -> d/q/1
  q/1 -> Mux/2
  d/1 -> Mux/1

== system deneme/Inverter Control1/vdq - Vabc/alfa//beta - abc ==
  alfa/beta : Inport
  Mux : Mux  Inputs=3
  a : Fcn  Expr=u[2]
  b : Fcn  Expr=-sqrt(3)/2*u[1]-0.5*u[2]
  c : Fcn  Expr=sqrt(3)/2*u[1]-0.5*u[2]
  abc : Outport
  tag scope: Vca_ref2=global, Vcb_ref2=global, Vcc_ref2=global
  wires:
  alfa/beta/1 -> c/1, a/1, b/1
  Mux/1 -> abc/1
  c/1 -> Mux/3, [Vcc_ref2]
  b/1 -> Mux/2, [Vcb_ref2]
  a/1 -> Mux/1, [Vca_ref2]

== system deneme/Inverter Control1/vdq - Vabc/d//q - alfa//beta ==
  d/q : Inport
  tita : Inport  Port=2
  Mux : Mux  Inputs=2
  Mux1 : Mux  Inputs=2
  a : Fcn  Expr=-u[2]*sin(u[3]) + u[1]*cos(u[3])
  b : Fcn  Expr=u[1]*sin(u[3]) + u[2]*cos(u[3])
  alfa/beta : Outport
  wires:
  Mux1/1 -> b/1, a/1
  tita/1 -> Mux1/2
  d/q/1 -> Mux1/1
  a/1 -> Mux/1
  b/1 -> Mux/2
  Mux/1 -> alfa/beta/1

== system deneme/Inverter Control2/Iabc  - idq/abc  - alfa//beta ==
  abc : Inport
  Mux : Mux  Inputs=2
  d_s : Fcn  Expr=(-1/sqrt(3)*u(2))+(1/sqrt(3)*u(3))
  q_s : Fcn  Expr=(2/3)*u(1)-(1/3)*u(2)-(1/3)*u(3)
  alfa/beta : Outport
  wires:
  abc/1 -> q_s/1, d_s/1
  d_s/1 -> Mux/1
  q_s/1 -> Mux/2
  Mux/1 -> alfa/beta/1

== system deneme/Inverter Control2/Iabc  - idq/alfa//beta - dq ==
  alfa/beta : Inport
  theta : Inport  Port=2
  Mux : Mux  Inputs=2
  Mux1 : Mux  Inputs=2
  d : Fcn  Expr=u(2)*sin(u(3)) + u(1)*cos(u(3))
  q : Fcn  Expr=-u(1)*sin(u(3)) + u(2)*cos(u(3))
  d/q : Outport
  wires:
  d/1 -> Mux/1
  q/1 -> Mux/2
  Mux/1 -> d/q/1
  alfa/beta/1 -> Mux1/1
  theta/1 -> Mux1/2
  Mux1/1 -> d/1, q/1

== system deneme/Inverter Control2/Vabc  - vdq/abc  - alfa//beta ==
  abc : Inport
  Mux : Mux  Inputs=2
  d_s : Fcn  Expr=(-1/sqrt(3)*u(2))+(1/sqrt(3)*u(3))
  q_s : Fcn  Expr=(2/3)*u(1)-(1/3)*u(2)-(1/3)*u(3)
  alfa/beta : Outport
  wires:
  Mux/1 -> alfa/beta/1
  q_s/1 -> Mux/2
  d_s/1 -> Mux/1
  abc/1 -> d_s/1, q_s/1

== system deneme/Inverter Control2/Vabc  - vdq/alfa//beta - dq ==
  alfa/beta : Inport
  theta : Inport  Port=2
  Mux : Mux  Inputs=2
  Mux1 : Mux  Inputs=2
  d : Fcn  Expr=u(2)*sin(u(3)) + u(1)*cos(u(3))
  q : Fcn  Expr=-u(1)*sin(u(3)) + u(2)*cos(u(3))
  d/q : Outport
  wires:
  Mux1/1 -> q/1, d/1
  theta/1 -> Mux1/2
  alfa/beta/1 -> Mux1/1
  Mux/1 -> d/q/1
  q/1 -> Mux/2
  d/1 -> Mux/1

== system deneme/Inverter Control2/vdq - Vabc/alfa//beta - abc ==
  alfa/beta : Inport
  Mux : Mux  Inputs=3
  a : Fcn  Expr=u[2]
  b : Fcn  Expr=-sqrt(3)/2*u[1]-0.5*u[2]
  c : Fcn  Expr=sqrt(3)/2*u[1]-0.5*u[2]
  abc : Outport
  tag scope: Vca_ref3=global, Vcb_ref3=global, Vcc_ref3=global
  wires:
  alfa/beta/1 -> c/1, a/1, b/1
  Mux/1 -> abc/1
  c/1 -> Mux/3, [Vcc_ref3]
  b/1 -> Mux/2, [Vcb_ref3]
  a/1 -> Mux/1, [Vca_ref3]

== system deneme/Inverter Control2/vdq - Vabc/d//q - alfa//beta ==
  d/q : Inport
  tita : Inport  Port=2
  Mux : Mux  Inputs=2
  Mux1 : Mux  Inputs=2
  a : Fcn  Expr=-u[2]*sin(u[3]) + u[1]*cos(u[3])
  b : Fcn  Expr=u[1]*sin(u[3]) + u[2]*cos(u[3])
  alfa/beta : Outport
  wires:
  Mux1/1 -> b/1, a/1
  tita/1 -> Mux1/2
  d/q/1 -> Mux1/1
  a/1 -> Mux/1
  b/1 -> Mux/2
  Mux/1 -> alfa/beta/1

== system deneme/Subsystem/Inverter Control Measurements/Subsystem1 ==
  vd_ref : Inport
  To Workspace1 : ToWorkspace  VariableName=vd_ref  SampleTime=-1
  Zero-Order Hold1 : ZeroOrderHold  SampleTime=5e-6
  wires:
  vd_ref/1 -> Zero-Order Hold1/1
  Zero-Order Hold1/1 -> To Workspace1/1

== system deneme/Subsystem/Inverter Control Measurements/Subsystem10 ==
  f_ref : Inport
  To Workspace1 : ToWorkspace  VariableName=f_ref  SampleTime=-1
  Zero-Order Hold1 : ZeroOrderHold  SampleTime=5e-6
  wires:
  f_ref/1 -> Zero-Order Hold1/1
  Zero-Order Hold1/1 -> To Workspace1/1

== system deneme/Subsystem/Inverter Control Measurements/Subsystem11 ==
  theta : Inport
  To Workspace1 : ToWorkspace  VariableName=theta  SampleTime=-1
  Zero-Order Hold1 : ZeroOrderHold  SampleTime=5e-6
  wires:
  theta/1 -> Zero-Order Hold1/1
  Zero-Order Hold1/1 -> To Workspace1/1

== system deneme/Subsystem/Inverter Control Measurements/Subsystem12 ==
  m_index : Inport
  To Workspace1 : ToWorkspace  VariableName=m_index  SampleTime=-1
  Zero-Order Hold1 : ZeroOrderHold  SampleTime=5e-6
  wires:
  m_index/1 -> Zero-Order Hold1/1
  Zero-Order Hold1/1 -> To Workspace1/1

== system deneme/Subsystem/Inverter Control Measurements/Subsystem13 ==
  pulses : Inport
  To Workspace1 : ToWorkspace  VariableName=pulses  SampleTime=-1
  Zero-Order Hold1 : ZeroOrderHold  SampleTime=5e-6
  wires:
  pulses/1 -> Zero-Order Hold1/1
  Zero-Order Hold1/1 -> To Workspace1/1

== system deneme/Subsystem/Inverter Control Measurements/Subsystem2 ==
  vq_ref : Inport
  To Workspace1 : ToWorkspace  VariableName=vq_ref  SampleTime=-1
  Zero-Order Hold1 : ZeroOrderHold  SampleTime=5e-6
  wires:
  vq_ref/1 -> Zero-Order Hold1/1
  Zero-Order Hold1/1 -> To Workspace1/1

== system deneme/Subsystem/Inverter Control Measurements/Subsystem3 ==
  vd : Inport
  To Workspace1 : ToWorkspace  VariableName=vd  SampleTime=-1
  Zero-Order Hold1 : ZeroOrderHold  SampleTime=5e-6
  wires:
  vd/1 -> Zero-Order Hold1/1
  Zero-Order Hold1/1 -> To Workspace1/1

== system deneme/Subsystem/Inverter Control Measurements/Subsystem4 ==
  vq : Inport
  To Workspace1 : ToWorkspace  VariableName=vq  SampleTime=-1
  Zero-Order Hold1 : ZeroOrderHold  SampleTime=5e-6
  wires:
  vq/1 -> Zero-Order Hold1/1
  Zero-Order Hold1/1 -> To Workspace1/1

== system deneme/Subsystem/Inverter Control Measurements/Subsystem5 ==
  id_ref : Inport
  To Workspace1 : ToWorkspace  VariableName=id_ref  SampleTime=-1
  Zero-Order Hold1 : ZeroOrderHold  SampleTime=5e-6
  wires:
  id_ref/1 -> Zero-Order Hold1/1
  Zero-Order Hold1/1 -> To Workspace1/1

== system deneme/Subsystem/Inverter Control Measurements/Subsystem6 ==
  id : Inport
  To Workspace1 : ToWorkspace  VariableName=id  SampleTime=-1
  Zero-Order Hold1 : ZeroOrderHold  SampleTime=5e-6
  wires:
  id/1 -> Zero-Order Hold1/1
  Zero-Order Hold1/1 -> To Workspace1/1

== system deneme/Subsystem/Inverter Control Measurements/Subsystem7 ==
  iq_ref : Inport
  To Workspace1 : ToWorkspace  VariableName=iq_ref  SampleTime=-1
  Zero-Order Hold1 : ZeroOrderHold  SampleTime=5e-6
  wires:
  iq_ref/1 -> Zero-Order Hold1/1
  Zero-Order Hold1/1 -> To Workspace1/1

== system deneme/Subsystem/Inverter Control Measurements/Subsystem8 ==
  iq : Inport
  To Workspace1 : ToWorkspace  VariableName=iq  SampleTime=-1
  Zero-Order Hold1 : ZeroOrderHold  SampleTime=5e-6
  wires:
  iq/1 -> Zero-Order Hold1/1
  Zero-Order Hold1/1 -> To Workspace1/1

== system deneme/Subsystem/Inverter Control Measurements/Subsystem9 ==
  Vabc_ref : Inport
  To Workspace1 : ToWorkspace  VariableName=Vabc_ref  SampleTime=-1
  Zero-Order Hold1 : ZeroOrderHold  SampleTime=5e-6
  wires:
  Vabc_ref/1 -> Zero-Order Hold1/1
  Zero-Order Hold1/1 -> To Workspace1/1

== system deneme/Subsystem/Inverter Control Measurements3/PLL ==
  Vabc : Inport
  Demux : Demux  Outputs=2
  Integrator : Integrator
  PI : Subsystem
  Subsystem3 : Subsystem
  Terminator : Terminator
  abc  - d/q : Subsystem
  wires:
  Vabc/1 -> abc  - d/q/1(abc)
  Integrator/1 -> abc  - d/q/2(tita)
  PI/1(w) -> Integrator/1, Subsystem3/1(wabc)
  Demux/2 -> PI/1(e)
  abc  - d/q/1(d/q) -> Demux/1
  Demux/1 -> Terminator/1

== system deneme/Subsystem/Inverter Control Measurements3/Subsystem ==
  LPF vq2 : powerlib_extras/Discrete  Control Blocks/Discrete 1st-Order Filter  FilterType=Lowpass  Tc=10e-3  Ts=5e-6  Initialize=off  Vac_Init=[0.8 -25 60]  Vdc_Init=0  PlotResponse=off  param1=[1 100 0.1]
  LPF vq3 : powerlib_extras/Discrete  Control Blocks/Discrete 1st-Order Filter  FilterType=Lowpass  Tc=10e-3  Ts=5e-6  Initialize=off  Vac_Init=[0.8 -25 60]  Vdc_Init=0  PlotResponse=off  param1=[1 100 0.1]
  LPF vq4 : powerlib_extras/Discrete  Control Blocks/Discrete 1st-Order Filter  FilterType=Lowpass  Tc=10e-3  Ts=5e-6  Initialize=off  Vac_Init=[0.8 -25 60]  Vdc_Init=0  PlotResponse=off  param1=[1 100 0.1]
  Mux : Mux  Inputs=3
  Vabc : Outport
  wires:
  [Vab] -> LPF vq2/1
  [Vbc] -> LPF vq3/1
  [Vca] -> LPF vq4/1
  LPF vq2/1 -> Mux/1
  LPF vq3/1 -> Mux/2
  LPF vq4/1 -> Mux/3
  Mux/1 -> Vabc/1

== system deneme/Subsystem/Load Power Calculation/Subsystem1 ==
  Qacload : Inport
  LPF vq7 : powerlib_extras/Discrete  Control Blocks/Discrete 1st-Order Filter  FilterType=Lowpass  Tc=10e-3  Ts=5e-6  Initialize=off  Vac_Init=[0.8 -25 60]  Vdc_Init=0  PlotResponse=off  param1=[1 100 0.1]
  To Workspace1 : ToWorkspace  VariableName=Qacload  SampleTime=-1
  To Workspace2 : ToWorkspace  VariableName=Qacload1  SampleTime=-1
  Zero-Order Hold : ZeroOrderHold  SampleTime=5e-6
  tag scope: Qacload=global
  wires:
  Qacload/1 -> Zero-Order Hold/1
  Zero-Order Hold/1 -> [Qacload], To Workspace2/1, LPF vq7/1
  LPF vq7/1 -> To Workspace1/1

== system deneme/Subsystem/Load Power Calculation/Subsystem2 ==
  Pload : Inport
  LPF vq7 : powerlib_extras/Discrete  Control Blocks/Discrete 1st-Order Filter  FilterType=Lowpass  Tc=10e-3  Ts=5e-6  Initialize=off  Vac_Init=[0.8 -25 60]  Vdc_Init=0  PlotResponse=off  param1=[1 100 0.1]
  To Workspace1 : ToWorkspace  VariableName=Pacload  SampleTime=-1
  To Workspace2 : ToWorkspace  VariableName=Pacload1  SampleTime=-1
  Zero-Order Hold : ZeroOrderHold  SampleTime=5e-6
  tag scope: Pacload=global
  wires:
  Pload/1 -> Zero-Order Hold/1
  Zero-Order Hold/1 -> [Pacload], To Workspace2/1, LPF vq7/1
  LPF vq7/1 -> To Workspace1/1

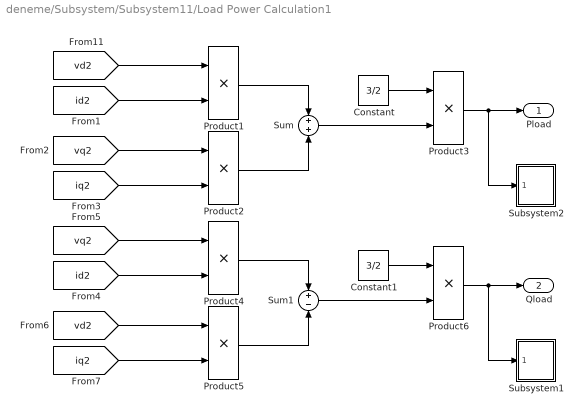
== system deneme/Subsystem/Subsystem11/Load Power Calculation1 ==
  Constant : Constant  Value=3/2
  Constant1 : Constant  Value=3/2
  Product{1..6} (6 alike) : Product  RndMeth=Zero
  Subsystem1 : Subsystem
  Subsystem2 : Subsystem
  Sum : Sum  Inputs=+|+
  Sum1 : Sum  Inputs=+|-
  Pload : Outport
  Qload : Outport  Port=2
  wires:
  Product6/1 -> Qload/1, Subsystem1/1(Qacload)
  Constant1/1 -> Product6/1
  Sum1/1 -> Product6/2
  Product5/1 -> Sum1/2
  Product4/1 -> Sum1/1
  [iq2] -> Product5/2
  [vd2] -> Product5/1
  [id2] -> Product4/2
  [vq2] -> Product4/1
  Product3/1 -> Pload/1, Subsystem2/1(Pload)
  Constant/1 -> Product3/1
  Sum/1 -> Product3/2
  Product2/1 -> Sum/2
  Product1/1 -> Sum/1
  [iq2] -> Product2/2
  [vq2] -> Product2/1
  [id2] -> Product1/2
  [vd2] -> Product1/1

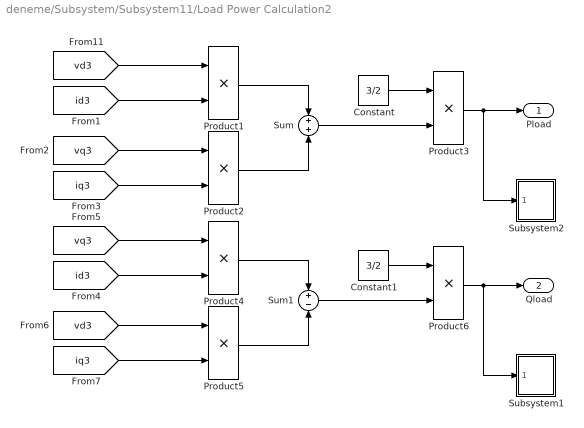
== system deneme/Subsystem/Subsystem11/Load Power Calculation2 ==
  Constant : Constant  Value=3/2
  Constant1 : Constant  Value=3/2
  Product{1..6} (6 alike) : Product  RndMeth=Zero
  Subsystem1 : Subsystem
  Subsystem2 : Subsystem
  Sum : Sum  Inputs=+|+
  Sum1 : Sum  Inputs=+|-
  Pload : Outport
  Qload : Outport  Port=2
  wires:
  [vd3] -> Product1/1
  [id3] -> Product1/2
  [vq3] -> Product2/1
  [iq3] -> Product2/2
  Product1/1 -> Sum/1
  Product2/1 -> Sum/2
  Sum/1 -> Product3/2
  Constant/1 -> Product3/1
  Product3/1 -> Pload/1, Subsystem2/1(Pload)
  [vq3] -> Product4/1
  [id3] -> Product4/2
  [vd3] -> Product5/1
  [iq3] -> Product5/2
  Product4/1 -> Sum1/1
  Product5/1 -> Sum1/2
  Sum1/1 -> Product6/2
  Constant1/1 -> Product6/1
  Product6/1 -> Qload/1, Subsystem1/1(Qacload)

== system deneme/Subsystem/Inverter Control Measurements3/PLL/PI ==
  e : Inport
  Gain1 : Gain  Gain=10
  Gain2 : Gain  Gain=100
  Integrator : Integrator
  Saturation : Saturate  UpperLimit=inf  LowerLimit=-inf
  Sum1 : Sum  Inputs=|++
  w : Outport
  wires:
  Integrator/1 -> Sum1/2
  Gain1/1 -> Sum1/1
  e/1 -> Gain2/1, Gain1/1
  Gain2/1 -> Integrator/1
  Saturation/1 -> w/1
  Sum1/1 -> Saturation/1

== system deneme/Subsystem/Inverter Control Measurements3/PLL/Subsystem3 ==
  wabc : Inport
  LPF vq7 : powerlib_extras/Discrete  Control Blocks/Discrete 1st-Order Filter  FilterType=Lowpass  Tc=10e-3  Ts=5e-6  Initialize=off  Vac_Init=[0.8 -25 60]  Vdc_Init=0  PlotResponse=off  param1=[1 100 0.1]
  To Workspace1 : ToWorkspace  VariableName=wabc_real  SampleTime=-1
  To Workspace2 : ToWorkspace  VariableName=wabc_real_fil  SampleTime=-1
  Zero-Order Hold : ZeroOrderHold  SampleTime=5e-6
  tag scope: w_abc=global
  wires:
  LPF vq7/1 -> To Workspace2/1
  wabc/1 -> Zero-Order Hold/1
  Zero-Order Hold/1 -> LPF vq7/1, To Workspace1/1, [w_abc]

== system deneme/Subsystem/Inverter Control Measurements3/PLL/abc  - d//q ==
  abc : Inport
  tita : Inport  Port=2
  abc  - alfa/beta : Subsystem
  alfa/beta - dq : Subsystem
  d/q : Outport
  wires:
  tita/1 -> alfa/beta - dq/2(tita)
  alfa/beta - dq/1(d/q) -> d/q/1
  abc/1 -> abc  - alfa/beta/1(abc)
  abc  - alfa/beta/1(alfa/beta) -> alfa/beta - dq/1(alfa/beta)

== system deneme/Subsystem/Subsystem11/Load Power Calculation1/Subsystem1 ==
  Qacload : Inport
  LPF vq7 : powerlib_extras/Discrete  Control Blocks/Discrete 1st-Order Filter  FilterType=Lowpass  Tc=10e-3  Ts=5e-6  Initialize=off  Vac_Init=[0.8 -25 60]  Vdc_Init=0  PlotResponse=off  param1=[1 100 0.1]
  To Workspace1 : ToWorkspace  VariableName=Qacload3  SampleTime=-1
  To Workspace2 : ToWorkspace  VariableName=Qacload_3  SampleTime=-1
  Zero-Order Hold : ZeroOrderHold  SampleTime=5e-6
  tag scope: Qacload3=global
  wires:
  Qacload/1 -> Zero-Order Hold/1
  Zero-Order Hold/1 -> [Qacload3], To Workspace2/1, LPF vq7/1
  LPF vq7/1 -> To Workspace1/1

== system deneme/Subsystem/Subsystem11/Load Power Calculation1/Subsystem2 ==
  Pload : Inport
  LPF vq7 : powerlib_extras/Discrete  Control Blocks/Discrete 1st-Order Filter  FilterType=Lowpass  Tc=10e-3  Ts=5e-6  Initialize=off  Vac_Init=[0.8 -25 60]  Vdc_Init=0  PlotResponse=off  param1=[1 100 0.1]
  To Workspace1 : ToWorkspace  VariableName=Pacload3  SampleTime=-1
  To Workspace2 : ToWorkspace  VariableName=Pacload_3  SampleTime=-1
  Zero-Order Hold : ZeroOrderHold  SampleTime=5e-6
  tag scope: Pacload3=global
  wires:
  Pload/1 -> Zero-Order Hold/1
  Zero-Order Hold/1 -> [Pacload3], To Workspace2/1, LPF vq7/1
  LPF vq7/1 -> To Workspace1/1

== system deneme/Subsystem/Subsystem11/Load Power Calculation2/Subsystem1 ==
  Qacload : Inport
  LPF vq7 : powerlib_extras/Discrete  Control Blocks/Discrete 1st-Order Filter  FilterType=Lowpass  Tc=10e-3  Ts=5e-6  Initialize=off  Vac_Init=[0.8 -25 60]  Vdc_Init=0  PlotResponse=off  param1=[1 100 0.1]
  To Workspace1 : ToWorkspace  VariableName=Qacload2  SampleTime=-1
  To Workspace2 : ToWorkspace  VariableName=Qacload_2  SampleTime=-1
  Zero-Order Hold : ZeroOrderHold  SampleTime=5e-6
  tag scope: Qacload2=global
  wires:
  Qacload/1 -> Zero-Order Hold/1
  Zero-Order Hold/1 -> [Qacload2], To Workspace2/1, LPF vq7/1
  LPF vq7/1 -> To Workspace1/1

== system deneme/Subsystem/Subsystem11/Load Power Calculation2/Subsystem2 ==
  Pload : Inport
  LPF vq7 : powerlib_extras/Discrete  Control Blocks/Discrete 1st-Order Filter  FilterType=Lowpass  Tc=10e-3  Ts=5e-6  Initialize=off  Vac_Init=[0.8 -25 60]  Vdc_Init=0  PlotResponse=off  param1=[1 100 0.1]
  To Workspace1 : ToWorkspace  VariableName=Pacload2  SampleTime=-1
  To Workspace2 : ToWorkspace  VariableName=Pacload_2  SampleTime=-1
  Zero-Order Hold : ZeroOrderHold  SampleTime=5e-6
  tag scope: Pacload2=global
  wires:
  Pload/1 -> Zero-Order Hold/1
  Zero-Order Hold/1 -> [Pacload2], To Workspace2/1, LPF vq7/1
  LPF vq7/1 -> To Workspace1/1

== system deneme/Subsystem/Inverter Control Measurements3/PLL/abc  - d//q/abc  - alfa//beta ==
  abc : Inport
  Mux : Mux  Inputs=2
  d_s : Fcn  Expr=(-1/sqrt(3)*u[2])+(1/sqrt(3)*u[3])
  q_s : Fcn  Expr=(2/3)*u[1]-(1/3)*u[2]-(1/3)*u[3]
  alfa/beta : Outport
  wires:
  abc/1 -> q_s/1, d_s/1
  d_s/1 -> Mux/1
  q_s/1 -> Mux/2
  Mux/1 -> alfa/beta/1

== system deneme/Subsystem/Inverter Control Measurements3/PLL/abc  - d//q/alfa//beta - dq ==
  alfa/beta : Inport
  tita : Inport  Port=2
  Mux : Mux  Inputs=2
  Mux1 : Mux  Inputs=2
  d : Fcn  Expr=u[2]*sin(u[3]) + u[1]*cos(u[3])
  q : Fcn  Expr=-u[1]*sin(u[3]) + u[2]*cos(u[3])
  d/q : Outport
  wires:
  d/1 -> Mux/1
  q/1 -> Mux/2
  Mux/1 -> d/q/1
  alfa/beta/1 -> Mux1/1
  tita/1 -> Mux1/2
  Mux1/1 -> d/1, q/1

== matlab function deneme/Boost1/Incremental Conductance MPPT/MPPT IC ==
  data: delta output; Ipv input; Iprevious input; Vref output; Vpv input; Vprevious input; Vref_previous input; Ipv_prev_out output; Vpv_prev_out output
function [delta,Vref,Ipv_prev_out,Vpv_prev_out] = IncCond(Ipv,Iprevious,Vpv,Vprevious,Vref_previous)

% REFERENCE PAPERS:
% Trishan Esram, Patrick L. Chapman, "Comparison of Photovoltaic Array
% Maximum Power Tracking Techniques", IEEE Transactions on Energy
% COnversion, vol. 22, issue 2, June 2007.
%
% M. Lokanadham, K. Vijaya Bhaskar, "Incremental Conductance Based Maximum
% Power Point Tracking (MPPT) for Photovoltaic System" International
% Journal of Engineering Research and Applications (IJERA), vol. 2, issue
% 2, March-April 2012.


% The followoing code is an algorithm for a Maximum Power Point Tracking
% (MPPT) technique Incremental COnductance

Vbus = 600;

dI=Ipv-Iprevious;
dV=Vpv-Vprevious;

if (dV==0)
    if (dI==0)
        Vref=Vref_previous;
    else
        if (Ipv>0)
            Vref= Vpv+dV;
        else
            Vref= Vpv-dV;
        end
    end
else
    if ((dI/dV)==(-Ipv/Vpv))
        Vref=Vref_previous;
    else
        if ((dI/dV)>(-Ipv/Vpv))
            Vref= Vpv+dV;
        else
            Vref= Vpv-dV;
        end
    end
end
Ipv_prev_out=Ipv;
Vpv_prev_out=Vpv;

delta=1-Vref/Vbus;

end

== matlab function deneme/Boost2/Incremental Conductance MPPT/MPPT IC ==
  data: delta output; Ipv input; Iprevious input; Vref output; Vpv input; Vprevious input; Vref_previous input; Ipv_prev_out output; Vpv_prev_out output
function [delta,Vref,Ipv_prev_out,Vpv_prev_out] = IncCond(Ipv,Iprevious,Vpv,Vprevious,Vref_previous)

% REFERENCE PAPERS:
% Trishan Esram, Patrick L. Chapman, "Comparison of Photovoltaic Array
% Maximum Power Tracking Techniques", IEEE Transactions on Energy
% COnversion, vol. 22, issue 2, June 2007.
%
% M. Lokanadham, K. Vijaya Bhaskar, "Incremental Conductance Based Maximum
% Power Point Tracking (MPPT) for Photovoltaic System" International
% Journal of Engineering Research and Applications (IJERA), vol. 2, issue
% 2, March-April 2012.


% The followoing code is an algorithm for a Maximum Power Point Tracking
% (MPPT) technique Incremental COnductance

Vbus = 600;

dI=Ipv-Iprevious;
dV=Vpv-Vprevious;

if (dV==0)
    if (dI==0)
        Vref=Vref_previous;
    else
        if (Ipv>0)
            Vref= Vpv+dV;
        else
            Vref= Vpv-dV;
        end
    end
else
    if ((dI/dV)==(-Ipv/Vpv))
        Vref=Vref_previous;
    else
        if ((dI/dV)>(-Ipv/Vpv))
            Vref= Vpv+dV;
        else
            Vref= Vpv-dV;
        end
    end
end
Ipv_prev_out=Ipv;
Vpv_prev_out=Vpv;

delta=1-Vref/Vbus;

end
